simulink model "Simscape"  (R2021b)
(part 7 of 40)

  Joint3_Ring_Spacers_20_RIGID/LConn1 -- Transform77/RConn1
  Joint3_Ring_Spacers_26_RIGID/LConn1 -- Transform78/RConn1
  Transform7/RConn1 -- pan_cross_head_am_2_RIGID/LConn1
  Joint3_Ring_Spacers_28_RIGID/LConn1 -- Transform79/RConn1
  Joint3_Ring_Spacers_29_RIGID/LConn1 -- Transform80/RConn1
  Joint3_Ring_Spacers_30_RIGID/LConn1 -- Transform81/RConn1
  Joint3_Ring_Spacers_31_RIGID/LConn1 -- Transform82/RConn1
  Transform83/RConn1 -- pan_cross_head_am_20_RIGID/LConn1
  Transform84/RConn1 -- pan_cross_head_am_24_RIGID/LConn1
  Transform85/RConn1 -- pan_cross_head_am_11_RIGID/LConn1
  Transform86/RConn1 -- pan_cross_head_am_23_RIGID/LConn1
  Transform87/RConn1 -- pan_cross_head_am_7_RIGID/LConn1
  Transform88/RConn1 -- pan_cross_head_am_27_RIGID/LConn1
  Transform8/RConn1 -- pan_cross_head_am_3_RIGID/LConn1
  Transform89/RConn1 -- pan_cross_head_am_8_RIGID/LConn1
  Transform90/RConn1 -- pan_cross_head_am_12_RIGID/LConn1
  Transform91/RConn1 -- pan_cross_head_am_42_RIGID/LConn1
  Transform92/RConn1 -- pan_cross_head_am_10_RIGID/LConn1
  Transform93/RConn1 -- pan_cross_head_am_17_RIGID/LConn1
  Transform94/RConn1 -- pan_cross_head_am_6_RIGID/LConn1
  Transform95/RConn1 -- pan_cross_head_am_14_RIGID/LConn1
  Transform96/RConn1 -- pan_cross_head_am_15_RIGID/LConn1
  Transform97/RConn1 -- pan_cross_head_am_16_RIGID/LConn1
  Transform98/RConn1 -- pan_cross_head_am_18_RIGID/LConn1
